simulink model "Copy_of_mimo_malha_aberta"  (R2020a)
settings: Solver=VariableStepAuto  StartTime=0.0  StopTime=50000.0  RelTol=1e-3
libraries: cstblocks x8
settings Model: Creator=gabriel  LastModifiedBy=gabriel

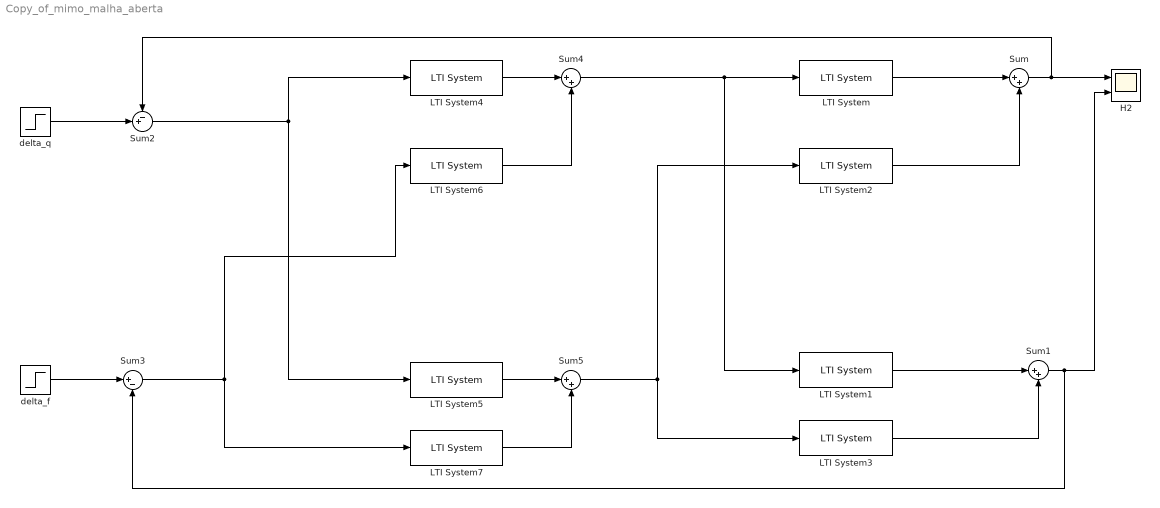
== system Copy_of_mimo_malha_aberta ==
  H2 : Scope  NumInputPorts=2
  LTI System : cstblocks/LTI System  sys=g11  IC=[]
  LTI System1 : cstblocks/LTI System  sys=g21  IC=[]
  LTI System2 : cstblocks/LTI System  sys=g12  IC=[]
  LTI System3 : cstblocks/LTI System  sys=g22  IC=[]
  LTI System4 : cstblocks/LTI System  sys=c11  IC=[]
  LTI System5 : cstblocks/LTI System  sys=c21  IC=[]
  LTI System6 : cstblocks/LTI System  sys=c12  IC=[]
  LTI System7 : cstblocks/LTI System  sys=c22  IC=[]
  Sum{,1,4..5} (4 alike) : Sum  Inputs=|++
  Sum2 : Sum  Inputs=-+|
  Sum3 : Sum  Inputs=|+-
  delta_f : Step  Time=20000  SampleTime=0
  delta_q : Step  SampleTime=0
  wires:
  LTI System3/1 -> Sum1/2
  LTI System/1 -> Sum/1
  Sum/1 -> Sum2/1, H2/1
  delta_q/1 -> Sum2/2
  delta_f/1 -> Sum3/1
  Sum1/1 -> Sum3/2, H2/2
  LTI System4/1 -> Sum4/1
  LTI System5/1 -> Sum5/1
  LTI System7/1 -> Sum5/2
  LTI System6/1 -> Sum4/2
  Sum5/1 -> LTI System3/1, LTI System2/1
  Sum4/1 -> LTI System/1, LTI System1/1
  Sum2/1 -> LTI System4/1, LTI System5/1
  Sum3/1 -> LTI System6/1, LTI System7/1
  LTI System1/1 -> Sum1/1
  LTI System2/1 -> Sum/2
